simulink model "E_DriveLab1AddTask"  (R2022a)
settings: Solver=ode3  StartTime=0.0  StopTime=250  FixedStep=1e-3  RelTol=1e-3
values from neighbouring files (symbols this model uses):
  B12 = ksi2*T2*2*K12    (= 14782.6516232)    [EDriveLab1.m]
  J1 = 1/Kw-J2    (= 76.7135019449)    [EDriveLab1.m]
  J2 = double(J_roots(2))    [EDriveLab1.m]
  K12 = J2/T1^2    (= 4345363.25052)    [EDriveLab1.m]
settings Model: Creator=Denis  LastModifiedBy=Family
settings DebuggingCC: UnconnectedInputMsg=warning  UnconnectedOutputMsg=warning  UnconnectedLineMsg=warning
settings RTWCC: DLArmComputeVersion=19.05

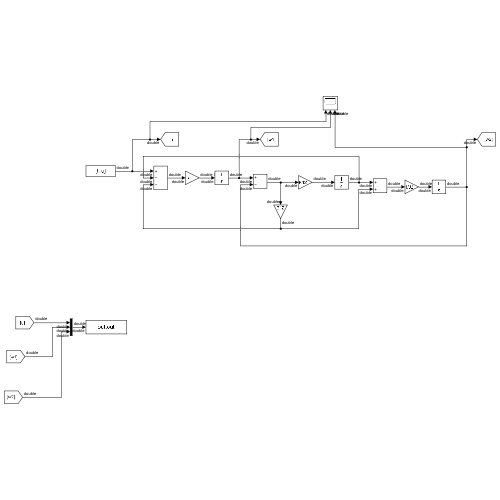
[thumbnail: Simulink's stored preview of the top-level diagram]
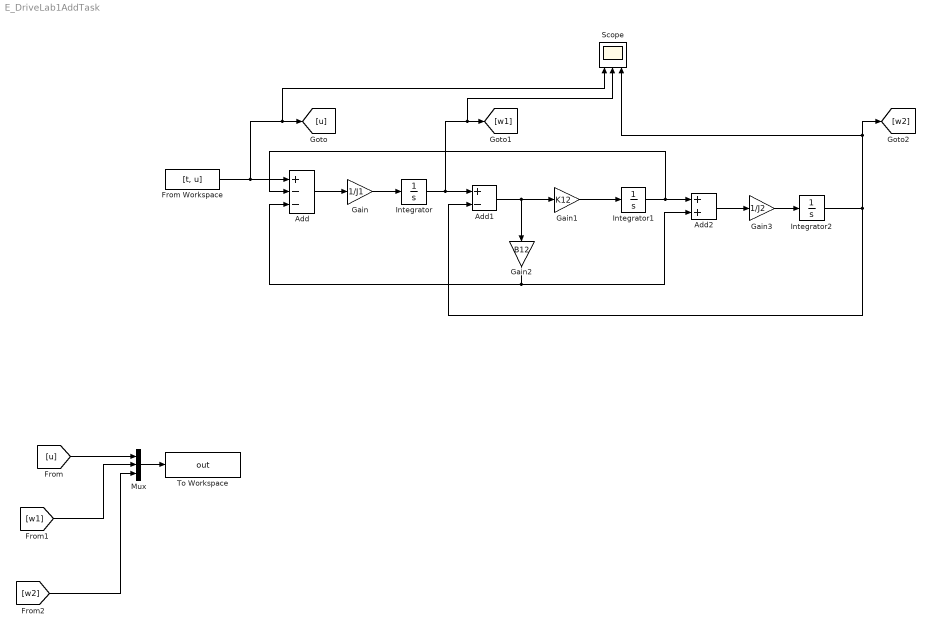
== system E_DriveLab1AddTask ==
  Add : Sum  Inputs=+--
  Add1 : Sum  Inputs=+-
  Add2 : Sum
  From Workspace : FromWorkspace  VariableName=[t, u]
  Gain : Gain  Gain=1/J1
  Gain1 : Gain  Gain=K12
  Gain2 : Gain  Gain=B12
  Gain3 : Gain  Gain=1/J2
  Integrator : Integrator
  Integrator1 : Integrator
  Integrator2 : Integrator
  Mux : Mux  Inputs=3
  Scope : Scope  NumInputPorts=3
  To Workspace : ToWorkspace  VariableName=out  SaveFormat=Structure With Time  SampleTime=-1
  wires:
  Integrator2/1 -> Scope/3, [w2], Add1/2
  Gain3/1 -> Integrator2/1
  Add2/1 -> Gain3/1
  Integrator1/1 -> Add/2, Add2/1
  Gain1/1 -> Integrator1/1
  Add1/1 -> Gain1/1, Gain2/1
  Integrator/1 -> Add1/1, Scope/2, [w1]
  From Workspace/1 -> Scope/1, [u], Add/1
  Add/1 -> Gain/1
  Gain/1 -> Integrator/1
  Gain2/1 -> Add2/2, Add/3
  [u] -> Mux/1
  [w1] -> Mux/2
  [w2] -> Mux/3
  Mux/1 -> To Workspace/1
